simulink model "sFunctionLibrary_q2dcm_Harness"  (R2025b)
settings: Solver=FixedStepAuto  StartTime=1  StopTime=15  FixedStep=1  RelTol=1e-3
settings Model: Creator=AdamY  LastModifiedBy=AdamY

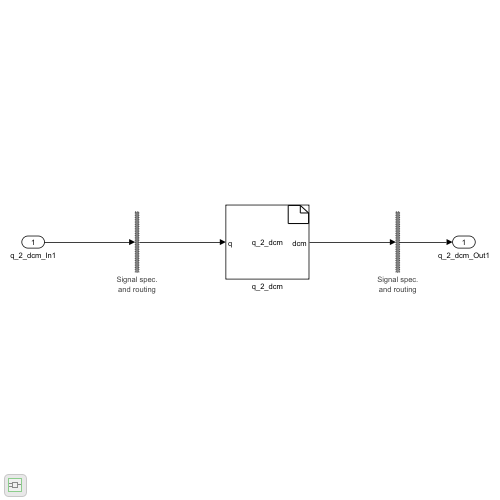
[thumbnail: Simulink's stored preview of the top-level diagram]
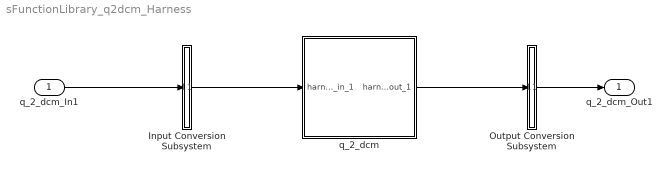
== system sFunctionLibrary_q2dcm_Harness ==
  q_2_dcm_In1 : Inport
  Input Conversion Subsystem : Subsystem  Tag=__SLT_ICS__  Description=|
      | Signal spec.
      | and routing
      settings: AttributesFormatString=%<Description>
  Output Conversion Subsystem : Subsystem  Tag=__SLT_OCS__  Description=|
      | Signal spec.
      | and routing
      settings: AttributesFormatString=%<Description>
  q_2_dcm : Subsystem  Tag=__SL_testing_harness_stub_
  q_2_dcm_Out1 : Outport
  wires:
  q_2_dcm_In1/1 -> Input Conversion Subsystem/1(Inport_1)
  Output Conversion Subsystem/1(Outport_1) -> q_2_dcm_Out1/1
  Input Conversion Subsystem/1(Outport_1) -> q_2_dcm/1(harness_in_1)
  q_2_dcm/1(harness_out_1) -> Output Conversion Subsystem/1(Inport_1)

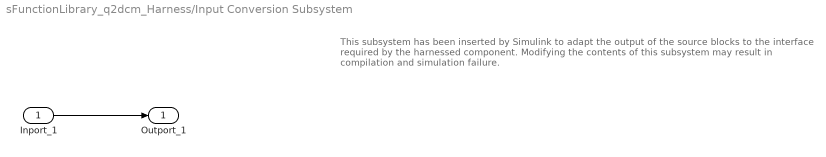
== system sFunctionLibrary_q2dcm_Harness/Input Conversion Subsystem ==
  note: This subsystem has been inserted by Simulink to adapt the output of the source blocks to the interface required by the harnessed component.
      |  Modifying the contents of this subsystem may result in compilation and simulation failure.
  Inport_1 : Inport
  Outport_1 : Outport
  wires:
  Inport_1/1 -> Outport_1/1

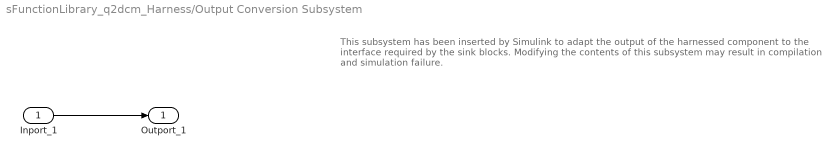
== system sFunctionLibrary_q2dcm_Harness/Output Conversion Subsystem ==
  note: This subsystem has been inserted by Simulink to adapt the output of the harnessed component to the interface required by the sink blocks.
      |  Modifying the contents of this subsystem may result in compilation and simulation failure.
  Inport_1 : Inport
  Outport_1 : Outport
  wires:
  Inport_1/1 -> Outport_1/1

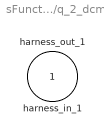
== system sFunctionLibrary_q2dcm_Harness/q_2_dcm ==
  harness_in_1 : Inport
  harness_out_1 : Outport
